simulink model "Adaptive_PID_2020b_new"  (R2020b)
settings: Solver=FixedStepAuto  StartTime=0.0  StopTime=60  FixedStep=0.01  RelTol=1e-3
undefined symbols (not defined in the file): DiscIntNeverNeededParam, LC_AdaptPID_a, LC_AdaptPID_b, LC_AdaptPID_Kd, LC_AdaptPID_Ki, LC_AdaptPID_Kp, LC_AdaptPID_mu_d, LC_AdaptPID_mu_i, LC_AdaptPID_mu_p
libraries: simulink x1
settings Model: Creator=Z0150218  LastModifiedBy=Z0150218
settings DebuggingCC: UnconnectedInputMsg=none  UnconnectedOutputMsg=none  UnconnectedLineMsg=none
settings ModelReferenceCC: EnableRefExpFcnMdlSchedulingChecks=off

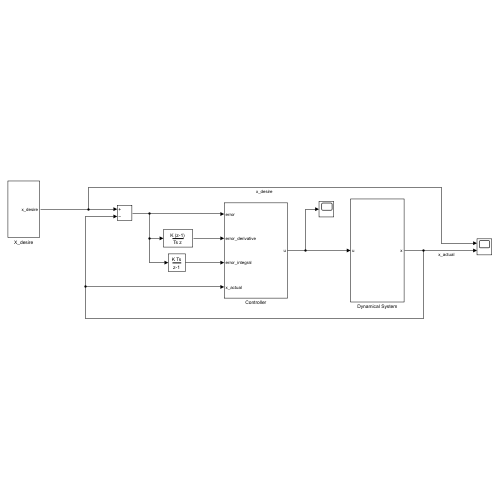
[thumbnail: Simulink's stored preview of the top-level diagram]
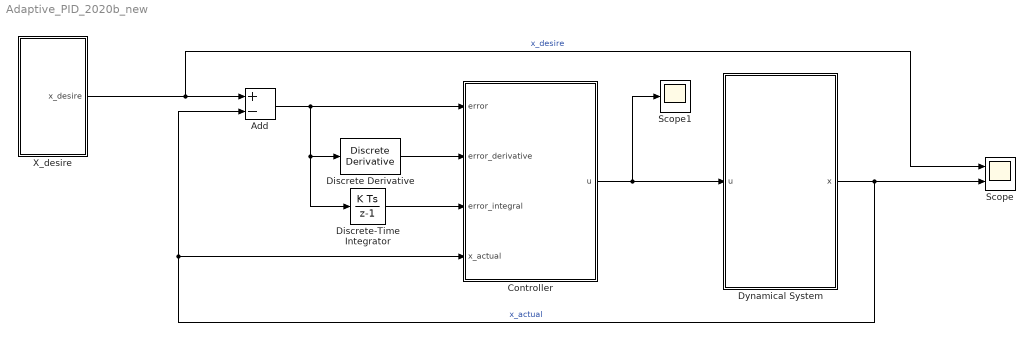
== system Adaptive_PID_2020b_new ==
  Add : Sum  Inputs=+-
  Controller : Subsystem
  Discrete Derivative : simulink/Discrete/Discrete Derivative  gainval=1.0  ICPrevScaledInput=0.0  OutMin=[]  OutMax=[]  OutDataType=fixdt(1, 16)  OutScaling=2^-10  DoSatur=off
  Discrete-Time Integrator : DiscreteIntegrator  SampleTime=-1  ICPrevOutput=DiscIntNeverNeededParam  ICPrevScaledInput=DiscIntNeverNeededParam
  Dynamical System : Subsystem
  Scope : Scope  NumInputPorts=2
  Scope1 : Scope
  X_desire : Subsystem
  wires:
  Dynamical System/1(x) -> Scope/2, Add/2, Controller/4(x_actual)  "x_actual"
  Controller/1(u) -> Scope1/1, Dynamical System/1(u)
  X_desire/1(x_desire) -> Scope/1, Add/1  "x_desire"
  Add/1 -> Discrete-Time Integrator/1, Discrete Derivative/1, Controller/1(error)
  Discrete Derivative/1 -> Controller/2(error_derivative)
  Discrete-Time Integrator/1 -> Controller/3(error_integral)

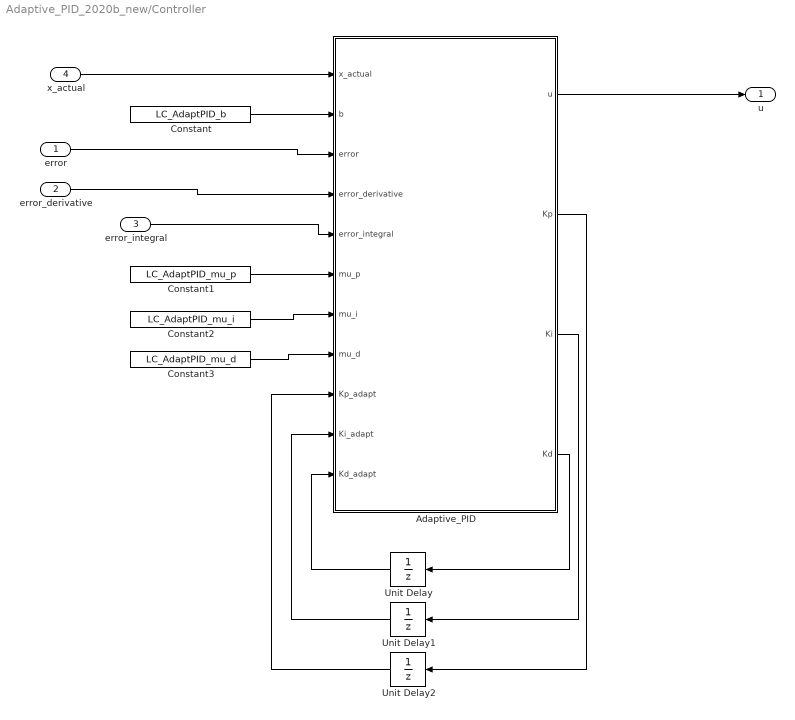
== system Adaptive_PID_2020b_new/Controller ==
  error : Inport
  error_derivative : Inport  Port=2
  error_integral : Inport  Port=3
  x_actual : Inport  Port=4
  Adaptive_PID : MATLAB Function  TreatAsAtomicUnit=on
  Constant : Constant  Value=LC_AdaptPID_b
  Constant1 : Constant  Value=LC_AdaptPID_mu_p
  Constant2 : Constant  Value=LC_AdaptPID_mu_i
  Constant3 : Constant  Value=LC_AdaptPID_mu_d
  Unit Delay : UnitDelay  InitialCondition=LC_AdaptPID_Kd  SampleTime=-1  HasFrameUpgradeWarning=on
  Unit Delay1 : UnitDelay  InitialCondition=LC_AdaptPID_Ki  SampleTime=-1  HasFrameUpgradeWarning=on
  Unit Delay2 : UnitDelay  InitialCondition=LC_AdaptPID_Kp  SampleTime=-1  HasFrameUpgradeWarning=on
  u : Outport
  wires:
  error_derivative/1 -> Adaptive_PID/4(error_derivative)
  Unit Delay1/1 -> Adaptive_PID/10(Ki_adapt)
  error/1 -> Adaptive_PID/3(error)
  Adaptive_PID/1(u) -> u/1
  Adaptive_PID/3(Ki) -> Unit Delay1/1
  Unit Delay/1 -> Adaptive_PID/11(Kd_adapt)
  error_integral/1 -> Adaptive_PID/5(error_integral)
  Constant/1 -> Adaptive_PID/2(b)
  Adaptive_PID/4(Kd) -> Unit Delay/1
  Adaptive_PID/2(Kp) -> Unit Delay2/1
  Unit Delay2/1 -> Adaptive_PID/9(Kp_adapt)
  x_actual/1 -> Adaptive_PID/1(x_actual)
  Constant1/1 -> Adaptive_PID/6(mu_p)
  Constant2/1 -> Adaptive_PID/7(mu_i)
  Constant3/1 -> Adaptive_PID/8(mu_d)

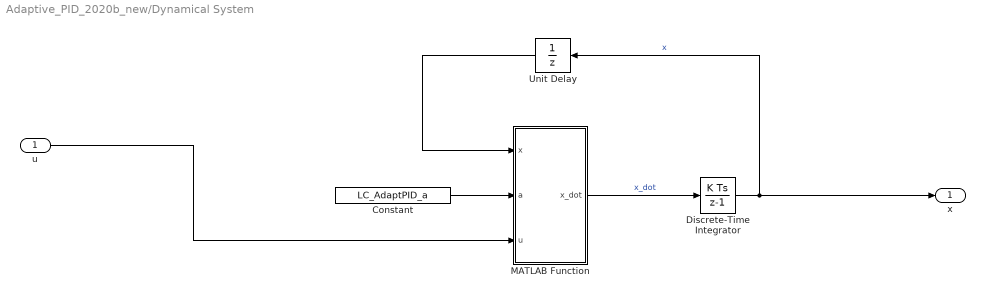
== system Adaptive_PID_2020b_new/Dynamical System ==
  u : Inport
  Constant : Constant  Value=LC_AdaptPID_a
  Discrete-Time Integrator : DiscreteIntegrator  SampleTime=-1  ICPrevOutput=DiscIntNeverNeededParam  ICPrevScaledInput=DiscIntNeverNeededParam
  MATLAB Function : MATLAB Function  TreatAsAtomicUnit=on
  Unit Delay : UnitDelay  SampleTime=-1  HasFrameUpgradeWarning=on
  x : Outport
  wires:
  Unit Delay/1 -> MATLAB Function/1(x)
  MATLAB Function/1(x_dot) -> Discrete-Time Integrator/1  "x_dot"
  Discrete-Time Integrator/1 -> x/1, Unit Delay/1  "x"
  Constant/1 -> MATLAB Function/2(a)
  u/1 -> MATLAB Function/3(u)

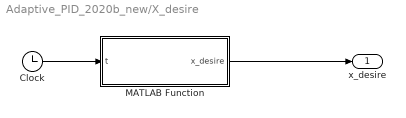
== system Adaptive_PID_2020b_new/X_desire ==
  Clock : Clock
  MATLAB Function : MATLAB Function  TreatAsAtomicUnit=on
  x_desire : Outport
  wires:
  Clock/1 -> MATLAB Function/1(t)
  MATLAB Function/1(x_desire) -> x_desire/1

== matlab function Adaptive_PID_2020b_new/X_desire/MATLAB Function ==
  data: t input; x_desire output
function x_desire = fcn(t)

if t < 5
    x_desire = 1;
else
    x_desire = sin(4 * t) * cos(3 * t); 
end 

end

== matlab function Adaptive_PID_2020b_new/Dynamical System/MATLAB Function ==
  data: x input; a input; u input; x_dot output
function x_dot = fcn(x,a,u)


x_dot = -a*(x^2) + u;

== matlab function Adaptive_PID_2020b_new/Controller/Adaptive_PID ==
  data: x_actual input; b input; u output; error input; error_derivative input; error_integral input; mu_p input; mu_i input; mu_d input; Kp output; Ki output; Kd output; Kp_adapt input; Ki_adapt input; Kd_adapt input
function [u,Kp,Ki,Kd] = fcn(x_actual,b,error, error_derivative, error_integral,mu_p,mu_i,mu_d,Kp_adapt,Ki_adapt,Kd_adapt) 


Kp = Kp_adapt + (mu_p * error * error);
Ki = Ki_adapt + (mu_i * error * error_integral);
Kd = Kd_adapt + (mu_d * error * error_derivative);


u = (Kp_adapt * error) + (Ki_adapt * error_integral) + (Kd_adapt * error_derivative) - (b*x_actual^2); 



end
